simulink model "rokubimini_serial_simulink"  (R2020b)
settings: Solver=VariableStepAuto  StartTime=0.0  StopTime=inf  RelTol=1e-3
undefined symbols (not defined in the file): serial
libraries: instrumentlib x3
settings Model: Creator=leftk  LastModifiedBy=leftk
settings DebuggingCC: InheritedTsInSrcMsg=none  UnderSpecifiedDimensionMsg=warning

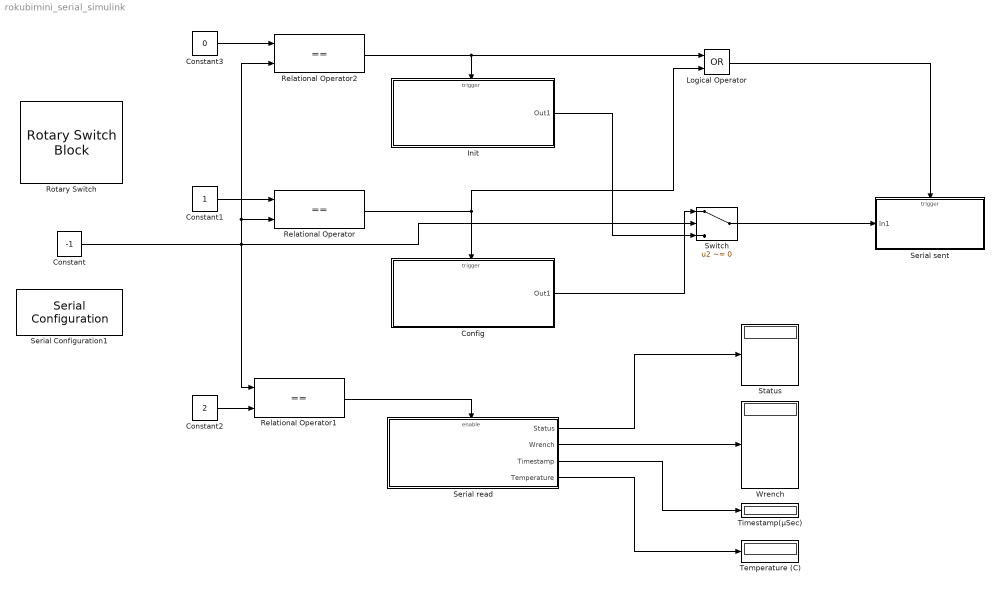
== system rokubimini_serial_simulink ==
  Config : Subsystem
  Constant : Constant  Value=-1
  Constant1 : Constant
  Constant2 : Constant  Value=2
  Constant3 : Constant  Value=0
  Init : Subsystem
  Logical Operator : Logic  Operator=OR  AllPortsSameDT=off  OutDataTypeStr=boolean
  Relational Operator : RelationalOperator  Operator===  OutDataTypeStr=boolean  RndMeth=Simplest
  Relational Operator1 : RelationalOperator  Operator===  OutDataTypeStr=boolean  RndMeth=Simplest
  Relational Operator2 : RelationalOperator  Operator===  OutDataTypeStr=boolean  RndMeth=Simplest
  Rotary Switch : RotarySwitchBlock
      settings: Values={{'Stop', 'Init', 'Config', 'Run'}, [-1 0 1 2]}
  Serial Configuration1 : instrumentlib/Serial Configuration  Priority=-200000  ComPortMenu=COM5  ComPort=COM5  ObjConstructor=serial('COM5');  BaudRate=460800  DataBits=8  Parity=none  StopBits=1  FlowControl=none  Timeout=10  ByteOrder=LittleEndian
  Serial read : Subsystem
  Serial sent : Subsystem
  Status : Display
  Switch : Switch  Criteria=u2 ~= 0
  Temperature (C) : Display
  Timestamp(μSec) : Display
  Wrench : Display
  wires:
  Serial read/1(Status) -> Status/1
  Serial read/2(Wrench) -> Wrench/1
  Serial read/3(Timestamp) -> Timestamp(μSec)/1
  Serial read/4(Temperature) -> Temperature (C)/1
  Constant/1 -> Relational Operator1/1, Switch/2, Relational Operator2/2, Relational Operator/2
  Constant1/1 -> Relational Operator/1
  Constant2/1 -> Relational Operator1/2
  Relational Operator1/1 -> Serial read/Enable
  Relational Operator/1 -> Logical Operator/2, Config/Trigger
  Constant3/1 -> Relational Operator2/1
  Relational Operator2/1 -> Init/Trigger, Logical Operator/1
  Switch/1 -> Serial sent/1(In1)
  Init/1(Out1) -> Switch/3
  Config/1(Out1) -> Switch/1
  Logical Operator/1 -> Serial sent/Trigger

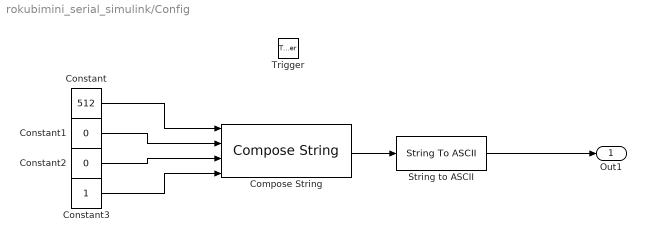
== system rokubimini_serial_simulink/Config ==
  Trigger : TriggerPort  VariantControl=Variant  PortDimensions=1
  Compose String : ComposeString  Format="\"Cf,%u,%u,%u,%uR\""
  Constant : Constant  Value=512  OutDataTypeStr=uint16  SampleTime=-1
  Constant1 : Constant  Value=0  OutDataTypeStr=uint8  SampleTime=-1
  Constant2 : Constant  Value=0  OutDataTypeStr=uint8  SampleTime=-1
  Constant3 : Constant  OutDataTypeStr=uint8  SampleTime=-1
  String to ASCII : StringToASCII  OutputVectorSize=16
  Out1 : Outport
  wires:
  Constant1/1 -> Compose String/2
  Constant3/1 -> Compose String/4
  Compose String/1 -> String to ASCII/1
  Constant/1 -> Compose String/1
  Constant2/1 -> Compose String/3
  String to ASCII/1 -> Out1/1

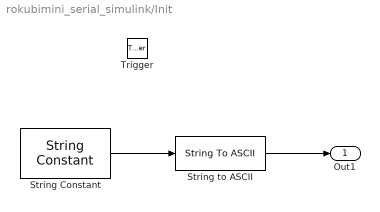
== system rokubimini_serial_simulink/Init ==
  Trigger : TriggerPort  VariantControl=Variant  PortDimensions=1
  String Constant : StringConstant  String="\"IR\""
  String to ASCII : StringToASCII  OutputVectorSize=16
  Out1 : Outport
  wires:
  String to ASCII/1 -> Out1/1
  String Constant/1 -> String to ASCII/1

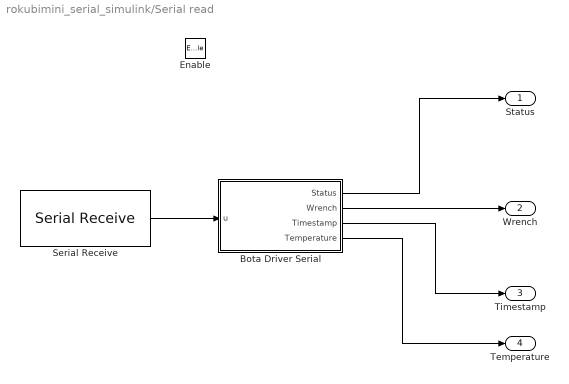
== system rokubimini_serial_simulink/Serial read ==
  Enable : EnablePort
  Bota Driver Serial : MATLAB Function  TreatAsAtomicUnit=on
  Serial Receive : instrumentlib/Serial Receive  ComPortMenu=COM5  ComPort=COM5  ObjConstructor=serial('COM5');  Header=ª  Terminator=<none>  DataSize="[36   1]"  DataType=uint8  EnableBlockingMode=on  ActionDataUnavailable=Output last received value  CustomValue=0  SampleTime=0.001
  Status : Outport
  Wrench : Outport  Port=2
  Timestamp : Outport  Port=3
  Temperature : Outport  Port=4
  wires:
  Serial Receive/1 -> Bota Driver Serial/1(u)
  Bota Driver Serial/4(Temperature) -> Temperature/1
  Bota Driver Serial/1(Status) -> Status/1
  Bota Driver Serial/3(Timestamp) -> Timestamp/1
  Bota Driver Serial/2(Wrench) -> Wrench/1

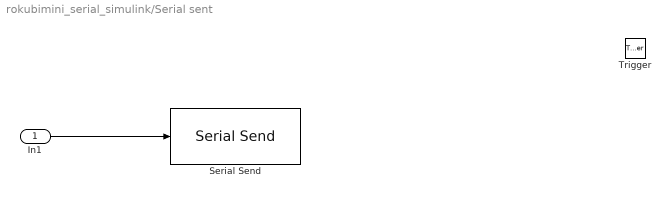
== system rokubimini_serial_simulink/Serial sent ==
  In1 : Inport
  Trigger : TriggerPort  VariantControl=Variant  PortDimensions=1
  Serial Send : instrumentlib/Serial Send  ComPortMenu=COM5  ComPort=COM5  ObjConstructor=serial('COM5');  Terminator=<none>  EnableBlockingMode=on
  wires:
  In1/1 -> Serial Send/1

== matlab function rokubimini_serial_simulink/Serial read/Bota Driver Serial ==
  data: u input; Status output uint8; Wrench output; Timestamp output uint32; Temperature output single
function [Status, Wrench, Timestamp, Temperature]  = Serial(u)

Timestamp = uint32(0);
Temperature = single(0);
Wrench = zeros(6,1);

Status = de2bi(u(1),8);

Wrench(1) = (typecast(uint8(u(3:6)),'single'));
Wrench(2) = (typecast(uint8(u(7:10)),'single'));
Wrench(3) = (typecast(uint8(u(11:14)),'single'));
Wrench(4) = (typecast(uint8(u(15:18)),'single'));
Wrench(5) = (typecast(uint8(u(19:22)),'single'));
Wrench(6) = (typecast(uint8(u(23:26)),'single'));

Timestamp = (typecast(uint8(u(27:30)),'uint32'));

Temperature = (typecast(uint8(u(31:34)),'single'));

end
